simulink model "test_remoteCtrl"  (R2015a)
settings: Solver=ode45  StartTime=0.0  StopTime=inf  RelTol=1e-3
libraries: Joymex2_lib x1, CrazyFlie_lib x1
settings Model: Creator=rshu  LastModifiedBy=rshu

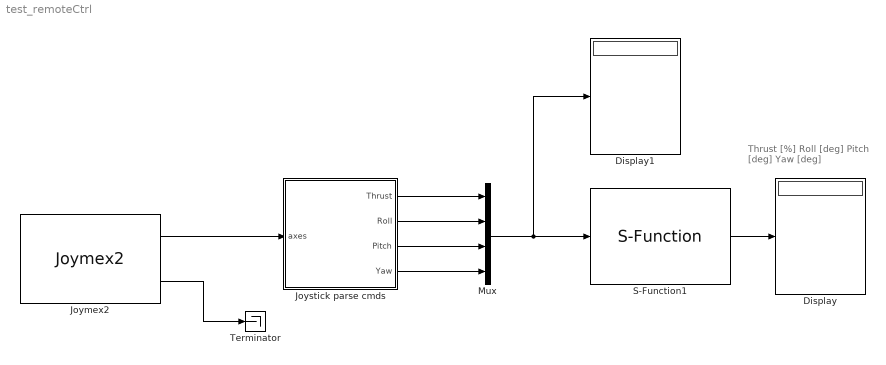
== system test_remoteCtrl ==
  note: Thrust [%]
      | Roll [deg]
      | Pitch [deg]
      | Yaw [deg]
  Display : Display
  Display1 : Display
  Joymex2 : Joymex2_lib/Joymex2
  Joystick parse cmds : Subsystem
  Mux : Mux
  S-Function1 : CrazyFlie_lib/S-Function
  Terminator : Terminator
  wires:
  S-Function1/1 -> Display/1
  Joymex2/2 -> Terminator/1
  Mux/1 -> S-Function1/1, Display1/1
  Joymex2/1 -> Joystick parse cmds/1(axes)
  Joystick parse cmds/1(Thrust) -> Mux/1
  Joystick parse cmds/2(Roll) -> Mux/2
  Joystick parse cmds/3(Pitch) -> Mux/3
  Joystick parse cmds/4(Yaw) -> Mux/4

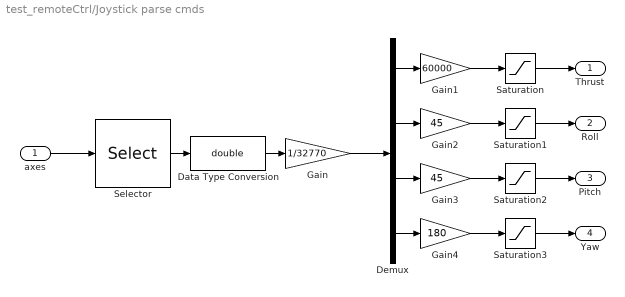
== system test_remoteCtrl/Joystick parse cmds ==
  axes : Inport
  Data Type Conversion : DataTypeConversion  OutDataTypeStr=double
  Demux : Demux
  Gain : Gain  Gain=1/32770
  Gain1 : Gain  Gain=60000
  Gain2 : Gain  Gain=45
  Gain3 : Gain  Gain=45
  Gain4 : Gain  Gain=180
  Saturation : Saturate  UpperLimit=60000  LowerLimit=9999
  Saturation1 : Saturate  UpperLimit=45  LowerLimit=-45
  Saturation2 : Saturate  UpperLimit=45  LowerLimit=-45
  Saturation3 : Saturate  UpperLimit=180  LowerLimit=-180
  Selector : Selector  InputPortWidth=7  Indices=[2 3 4 1]
  Thrust : Outport
  Roll : Outport  Port=2
  Pitch : Outport  Port=3
  Yaw : Outport  Port=4
  wires:
  Demux/2 -> Gain2/1
  Demux/1 -> Gain1/1
  axes/1 -> Selector/1
  Gain/1 -> Demux/1
  Demux/4 -> Gain4/1
  Data Type Conversion/1 -> Gain/1
  Demux/3 -> Gain3/1
  Selector/1 -> Data Type Conversion/1
  Gain1/1 -> Saturation/1
  Saturation/1 -> Thrust/1
  Saturation1/1 -> Roll/1
  Gain2/1 -> Saturation1/1
  Gain3/1 -> Saturation2/1
  Saturation2/1 -> Pitch/1
  Gain4/1 -> Saturation3/1
  Saturation3/1 -> Yaw/1
